simulink library "oneDoFGndStnCtrl_cl"  (R2018b)
settings: Solver=VariableStepAuto  StartTime=0.0  StopTime=10.0  RelTol=1e-3
settings Model: Creator=mcobb  LastModifiedBy=mcobb

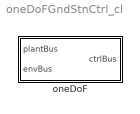
== system oneDoFGndStnCtrl_cl ==
  oneDoF : Subsystem

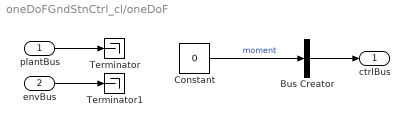
== system oneDoFGndStnCtrl_cl/oneDoF ==
  plantBus : Inport  OutDataTypeStr=Bus: plantBus
  envBus : Inport  Port=2  OutDataTypeStr=Bus: envBus
  Bus Creator : BusCreator  Inputs=1  OutDataTypeStr=Bus: gndStnCtrlBus
  Constant : Constant  Value=0
  Terminator : Terminator
  Terminator1 : Terminator
  ctrlBus : Outport  OutDataTypeStr=Bus: gndStnCtrlBus
  wires:
  Constant/1 -> Bus Creator/1  "moment"
  Bus Creator/1 -> ctrlBus/1
  plantBus/1 -> Terminator/1
  envBus/1 -> Terminator1/1
